simulink model "Hinf_DOB_MSD_LMI_sim"  (R2020b)
settings: Solver=VariableStepAuto  StartTime=0.0  StopTime=10.0  RelTol=1e-3
values from neighbouring files (symbols this model uses):
  A = [A0 b zeros(n0,1);zeros(1,n0) 0 0; zeros(1,n0) 0 Aa]    [DOB_MSD_LMI_Ptn1.m]    (also in DOB_MSD_poleplace.m = [A0 b ;zeros(1,n0) 0]; Hinf_DOB_MSD_LMI.m)
  B2 = [b;0;0]    [DOB_MSD_LMI_Ptn1.m]    (also in Hinf_DOB_MSD_LMI.m)
  C2 = [c 0 ca]    [DOB_MSD_LMI_Ptn1.m]    (also in Hinf_DOB_MSD_LMI.m)
  F = -D12_dag*C1    [DOB_MSD_LMI_Ptn1.m]    (also in Hinf_DOB_MSD_LMI.m)
  L = inv(U1) * inv(Y_U_a)*N_a    [DOB_MSD_LMI_Ptn1.m]    (also in DOB_MSD_poleplace.m = -place(A',C',p)'; Hinf_DOB_MSD_LMI.m)
libraries: cstblocks x2
settings Model: Creator=s0612  LastModifiedBy=s0612

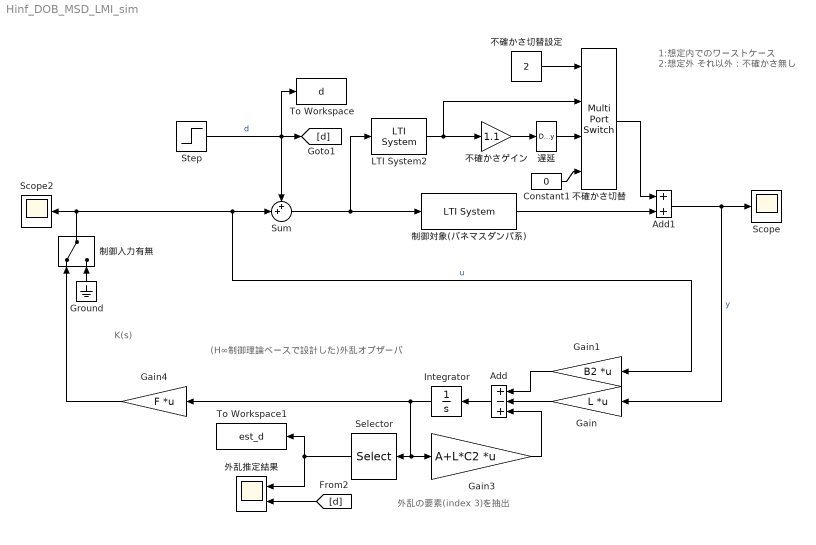
== system Hinf_DOB_MSD_LMI_sim ==
  note: K(s)
  note: 外乱の要素(index 3)を抽出
  note: 1:想定内でのワーストケース
      | 2:想定外
      | それ以外：不確かさ無し
  note: (H∞制御理論ベースで設計した)外乱オブザーバ
  Add : Sum  Inputs=+-+
  Add1 : Sum
  Constant1 : Constant  Value=0
  Gain : Gain  Gain=L  Multiplication=Matrix(K*u) (u vector)
  Gain1 : Gain  Gain=B2  Multiplication=Matrix(K*u) (u vector)
  Gain3 : Gain  Gain=A+L*C2  Multiplication=Matrix(K*u) (u vector)
  Gain4 : Gain  Gain=F  Multiplication=Matrix(K*u) (u vector)
  Ground : Ground
  Integrator : Integrator
  LTI System2 : cstblocks/LTI System  sys=Wa  IC=[]
  Scope : Scope
  Scope2 : Scope
  Selector : Selector  InputPortWidth=n  IndexOptions=Index vector (dialog)  Indices=[3]  OutputSizes=1
  Step : Step  SampleTime=0
  Sum : Sum  Inputs=++|
  To Workspace : ToWorkspace  VariableName=d  SaveFormat=Timeseries  SampleTime=-1
  To Workspace1 : ToWorkspace  VariableName=est_d  SaveFormat=Timeseries  SampleTime=-1
  不確かさゲイン : Gain  Gain=1.1
  不確かさ切替 : MultiPortSwitch  DiagnosticForDefault=None
  不確かさ切替設定 : Constant  Value=2
  制御入力有無 : ManualSwitch
  制御対象(バネマスダンパ系) : cstblocks/LTI System  sys=P  IC=[]
  外乱推定結果 : Scope  NumInputPorts=2
  遅延 : TransportDelay  DelayTime=5
  wires:
  Add1/1 -> Scope/1, Gain/1  "y"
  Sum/1 -> LTI System2/1, 制御対象(バネマスダンパ系)/1
  Step/1 -> To Workspace/1, [d], Sum/1  "d"
  制御入力有無/1 -> Sum/2, Gain1/1, Scope2/1  "u"
  Add/1 -> Integrator/1
  Gain/1 -> Add/2
  Integrator/1 -> Gain4/1, Gain3/1, Selector/1
  Selector/1 -> 外乱推定結果/1, To Workspace1/1
  Gain3/1 -> Add/3
  Gain1/1 -> Add/1
  [d] -> 外乱推定結果/2
  制御対象(バネマスダンパ系)/1 -> Add1/2
  不確かさ切替/1 -> Add1/1
  LTI System2/1 -> 不確かさ切替/2, 不確かさゲイン/1
  不確かさ切替設定/1 -> 不確かさ切替/1
  不確かさゲイン/1 -> 遅延/1
  Constant1/1 -> 不確かさ切替/4
  Gain4/1 -> 制御入力有無/1
  Ground/1 -> 制御入力有無/2
  遅延/1 -> 不確かさ切替/3
